simulink model "excitable_cell"  (R2021a)
settings: Solver=FixedStepAuto  StartTime=0.0  StopTime=timeFinal  FixedStep=timeStepMax  MaxStep=timeStepMax  RelTol=1e-3
model workspace (MAT data in the model file):
  x0 = 5
  y0 = 5
settings Model: SimulationMode=accelerator  Creator=amit  LastModifiedBy=amit
settings DataIOCC: ExternalInput=ds

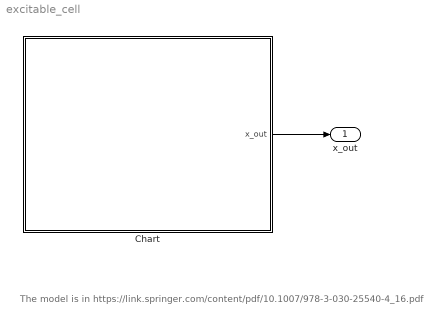
== system excitable_cell ==
  note: The model is in https://link.springer.com/content/pdf/10.1007/978-3-030-25540-4_16.pdf
  Chart : Stateflow chart  TreatAsAtomicUnit=on
  x_out : Outport  SignalName=xOut
  wires:
  Chart/1(x_out) -> x_out/1

== stateflow chart excitable_cell/Chart ==
  settings: updateMethod=CONTINUOUS  executeAtInitialization=1
  state Early_Repolarization
    du:  % derivatives
    x_dot = -1.52;
    exit:
    x_out=x;
  state Plateau
    du:  % derivatives
    x_dot = -0.76;
    exit:
    x_out=x;
  state Upstroke
    du:  % derivatives
    x_dot = 130.02;
    exit:
    x_out=x;
  state Stimulate_Resting
    du:  % derivatives
    x_dot = 0.0;
    exit:
    x_out=x;
  state Final_Repolarization
    du:  % derivatives
    x_dot = -2.13;
    exit:
    x_out=x;
  Early_Repolarization -> Plateau [order 1] : [x >= 34 & x <= 36]{x=x;}
  Early_Repolarization -> Early_Repolarization [order 2] : [x>=34 & x<=46]{x=x;}
  Upstroke -> Early_Repolarization [order 1] : [x >= 44 & x <= 46]{x=x;}
  Plateau -> Final_Repolarization [order 1] : [x >= -6 & x <= -4]{x=x;}
  Plateau -> Plateau [order 2] : [x>=-6 & x<=36]{x=x;}
  Upstroke -> Upstroke [order 2] : [x>=-76 & x<=46]{x=x;}
  Stimulate_Resting -> Upstroke [order 1] : [x >= -76 & x <= -74]{x=x;}
  (default) -> Stimulate_Resting : {x=a0;}
  Final_Repolarization -> Stimulate_Resting [order 1] : [x >= -76 & x <= -74]{x=x;}
  Final_Repolarization -> Final_Repolarization [order 2] : [x>=-76 & x<=36]{x=x;}
  Stimulate_Resting -> Stimulate_Resting [order 2] : [x>=-76 & x<=-74]{x=x;}
  data: x_out output; x local double; a0 parameter
  data x settings: updateMethod=SF_CONTINUOUS_TIME_DATA
